simulink model "derivador_purot_digital"  (R2019b)
settings: Solver=VariableStepAuto  StartTime=0.0  StopTime=2  RelTol=1e-3
settings Model: Creator=fernandopassold  LastModifiedBy=fernandopassold
settings DataIOCC: ReturnWorkspaceOutputs=off
settings DebuggingCC: ArithmeticOperatorsInVariantConditions=warning
settings SFSimCC: SimUseLocalCustomCode=off  CustomCodeUndefinedFunction=UseInterfaceOnly
settings RTWCC: RTWUseLocalCustomCode=off

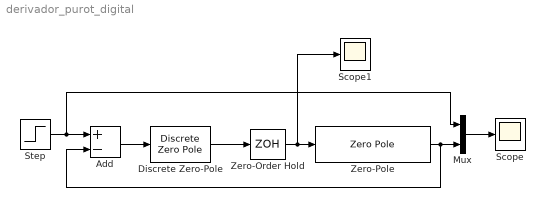
== system derivador_purot_digital ==
  Add : Sum  Inputs=+-
  Discrete Zero-Pole : DiscreteZeroPole  Poles=[0]  Gain=1  SampleTime=0.1
  Mux : Mux  Inputs=2
  Scope : Scope
  Scope1 : Scope
  Step : Step  SampleTime=0
  Zero-Order Hold : ZeroOrderHold  SampleTime=0.1
  Zero-Pole : ZeroPole  Zeros=[ ]  Poles=[-1 -2 -10]
  wires:
  Step/1 -> Mux/1, Add/1
  Mux/1 -> Scope/1
  Zero-Pole/1 -> Add/2, Mux/2
  Discrete Zero-Pole/1 -> Zero-Order Hold/1
  Zero-Order Hold/1 -> Scope1/1, Zero-Pole/1
  Add/1 -> Discrete Zero-Pole/1
